simulink model "Simulink_Simulation"  (R2022b)
settings: Solver=FixedStepAuto  StartTime=0.0  StopTime=30  FixedStep=5e-4  RelTol=1e-3
values from neighbouring files (symbols this model uses):
  Kd_PitchRate_val = 2    [Simscape_Simulation_Init.m]
  Kd_RollRate_val = 3    [Simscape_Simulation_Init.m]
  Kd_YawRate_val = 0e6    (= 0)    [Simscape_Simulation_Init.m]
  Ki_PitchRate_val = 7    [Simscape_Simulation_Init.m]
  Ki_RollRate_val = 7    [Simscape_Simulation_Init.m]
  Ki_Thrust_val = 200e6    (= 200000000)    [Simscape_Simulation_Init.m]
  Ki_YawRate_val = 100e6    (= 100000000)    [Simscape_Simulation_Init.m]
  Kp_PitchRate_val = 20    [Simscape_Simulation_Init.m]
  Kp_RollRate_val = 25    [Simscape_Simulation_Init.m]
  Kp_Thrust_val = 2e6    (= 2000000)    [Simscape_Simulation_Init.m]
  Kp_YawRate_val = 110e6    (= 110000000)    [Simscape_Simulation_Init.m]
  Kq_PitchRate_val = 4    [Simscape_Simulation_Init.m]
  Kr_YawRate_val = 7    [Simscape_Simulation_Init.m]
  N_PitchRate_val = 20    [Simscape_Simulation_Init.m]
  N_YawRate_val = 20    [Simscape_Simulation_Init.m]
  Ts_val = 0.01    [Simscape_Simulation_Init.m]
undefined symbols (not defined in the file or in its folder): DiscIntNeverNeededParam, smiData, X, Y, Z
libraries: sm_lib x27, nesl_utility x14, slpidlib x2, simulink x1
(part 1 of 2)
settings Model: Creator=marcv  LastModifiedBy=marcv

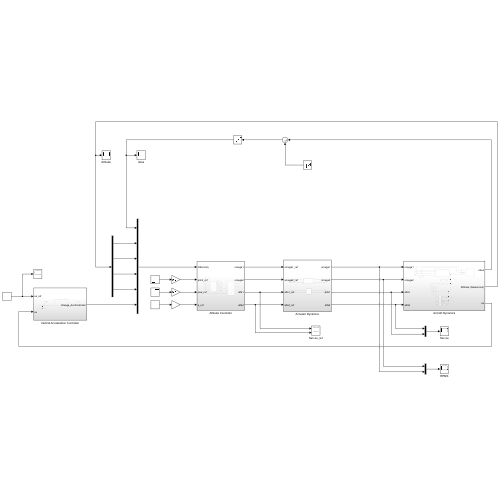
[thumbnail: Simulink's stored preview of the top-level diagram]
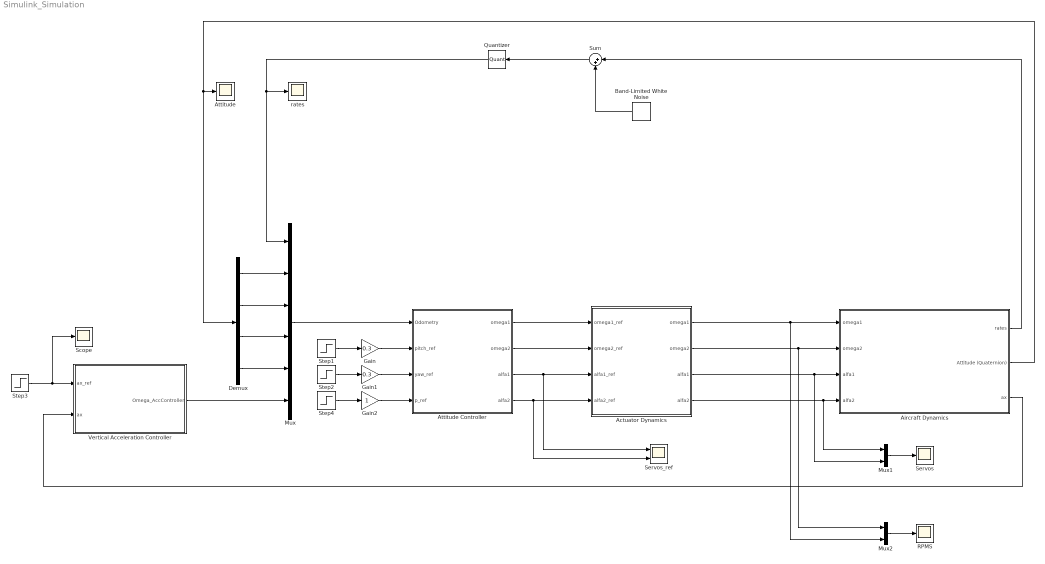
== system Simulink_Simulation ==
  Actuator Dynamics : Subsystem
  Aircraft Dynamics : Subsystem
  Attitude : Scope
  Attitude Controller : Subsystem
  Band-Limited White Noise : simulink/Sources/Band-Limited White Noise  Cov=[1e-6]  Ts=Ts_val  seed=[23341,43241,31231]
  Demux : Demux
  Gain : Gain  Gain=0.3
  Gain1 : Gain  Gain=0.3
  Gain2 : Gain
  Mux : Mux  Inputs=6
  Mux1 : Mux  Inputs=2
  Mux2 : Mux  Inputs=2
  Quantizer : Quantizer  QuantizationInterval=1e-3
  RPMS : Scope
  Scope : Scope
  Servos : Scope
  Servos_ref : Scope  NumInputPorts=2
  Step1 : Step  Time=10  SampleTime=0
  Step2 : Step  Time=10  SampleTime=0
  Step3 : Step  Before=2  After=2  SampleTime=0
  Step4 : Step  Time=10  SampleTime=0
  Sum : Sum  Inputs=|++
  Vertical Acceleration Controller : Subsystem
  rates : Scope
  wires:
  Mux/1 -> Attitude Controller/1(Odometry)
  Aircraft Dynamics/2(Attitude (Quaternion)) -> Demux/1, Attitude/1
  Aircraft Dynamics/3(ax) -> Vertical Acceleration Controller/2(ax)
  Step3/1 -> Scope/1, Vertical Acceleration Controller/1(ax_ref)
  Mux1/1 -> Servos/1
  Mux2/1 -> RPMS/1
  Vertical Acceleration Controller/1(Omega_AccController) -> Mux/6
  Demux/4 -> Mux/5
  Demux/3 -> Mux/4
  Demux/2 -> Mux/3
  Demux/1 -> Mux/2
  Gain/1 -> Attitude Controller/2(pitch_ref)
  Step1/1 -> Gain/1
  Step4/1 -> Gain2/1
  Step2/1 -> Gain1/1
  Gain1/1 -> Attitude Controller/3(yaw_ref)
  Gain2/1 -> Attitude Controller/4(p_ref)
  Actuator Dynamics/2(omega2) -> Aircraft Dynamics/2(omega2), Mux2/1
  Actuator Dynamics/3(alfa1) -> Mux1/2, Aircraft Dynamics/3(alfa1)
  Actuator Dynamics/4(alfa2) -> Mux1/1, Aircraft Dynamics/4(alfa2)
  Actuator Dynamics/1(omega1) -> Mux2/2, Aircraft Dynamics/1(omega1)
  Attitude Controller/1(omega1) -> Actuator Dynamics/1(omega1_ref)
  Attitude Controller/2(omega2) -> Actuator Dynamics/2(omega2_ref)
  Attitude Controller/3(alfa1) -> Actuator Dynamics/3(alfa1_ref), Servos_ref/1
  Attitude Controller/4(alfa2) -> Servos_ref/2, Actuator Dynamics/4(alfa2_ref)
  Quantizer/1 -> rates/1, Mux/1
  Aircraft Dynamics/1(rates) -> Sum/1
  Sum/1 -> Quantizer/1
  Band-Limited White Noise/1 -> Sum/2

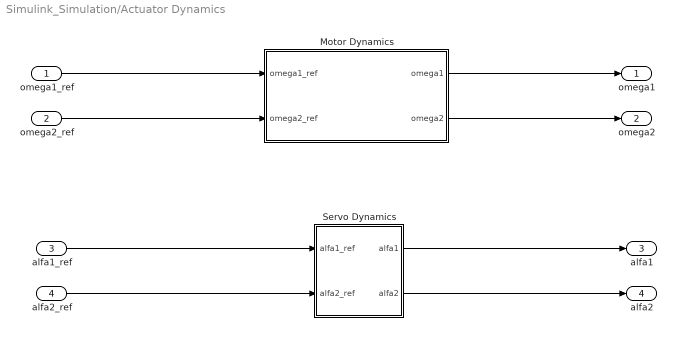
== system Simulink_Simulation/Actuator Dynamics ==
  omega1_ref : Inport
  omega2_ref : Inport  Port=2
  alfa1_ref : Inport  Port=3
  alfa2_ref : Inport  Port=4
  Motor Dynamics : Subsystem
  Servo Dynamics : Subsystem
  omega1 : Outport
  omega2 : Outport  Port=2
  alfa1 : Outport  Port=3
  alfa2 : Outport  Port=4
  wires:
  omega1_ref/1 -> Motor Dynamics/1(omega1_ref)
  alfa2_ref/1 -> Servo Dynamics/2(alfa2_ref)
  alfa1_ref/1 -> Servo Dynamics/1(alfa1_ref)
  omega2_ref/1 -> Motor Dynamics/2(omega2_ref)
  Servo Dynamics/1(alfa1) -> alfa1/1
  Servo Dynamics/2(alfa2) -> alfa2/1
  Motor Dynamics/1(omega1) -> omega1/1
  Motor Dynamics/2(omega2) -> omega2/1

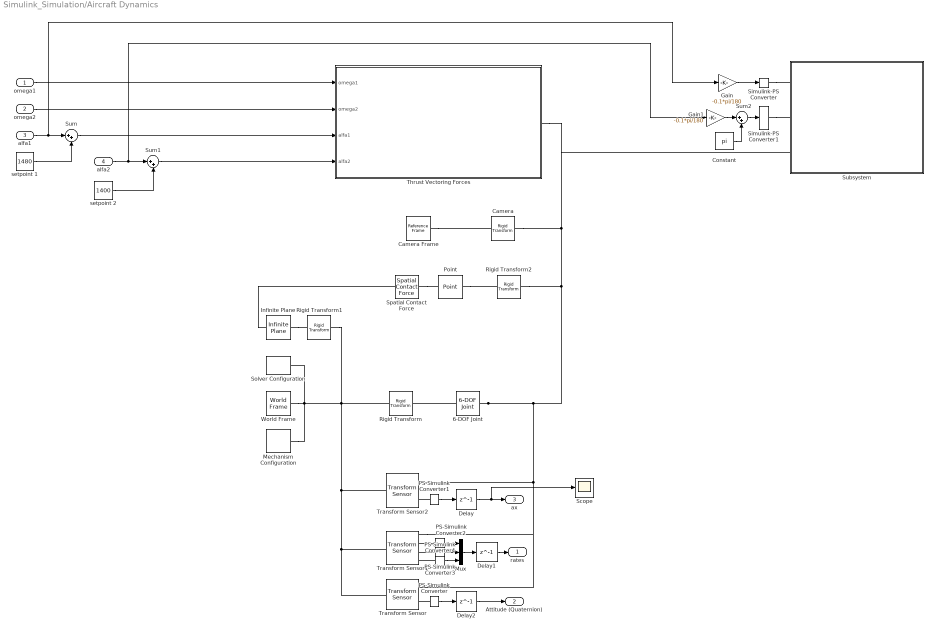
== system Simulink_Simulation/Aircraft Dynamics ==
  omega1 : Inport
  omega2 : Inport  Port=2
  alfa1 : Inport  Port=3
  alfa2 : Inport  Port=4
  6-DOF Joint : sm_lib/Joints/6-DOF Joint  JointMode=Normal  SenseConstraintForce=off  SenseConstraintForceX=off  SenseConstraintForceY=off  SenseConstraintForceZ=off  SenseConstraintTorque=off  SenseConstraintTorqueX=off  SenseConstraintTorqueY=off  SenseConstraintTorqueZ=off  SenseTotalForce=off  SenseTotalForceX=off  SenseTotalForceY=off  SenseTotalForceZ=off  SenseTotalTorque=off  SenseTotalTorqueX=off  SenseTotalTorqueY=off  SenseTotalTorqueZ=off  CompositeWrenchDir=FollowerOnBase  CompositeWrenchFrame=BaseFrame  PxEquilibriumPosition=0  PxEquilibriumPositionUnits=m  PxSpringStiffness=0  PxSpringStiffnessUnits=N/m  PxDampingCoefficient=0  PxDampingCoefficientUnits=N/(m/s)  PxTorqueActuationMode=NoTorque  PxMotionActuationMode=ComputedMotion  PxSensePosition=off  PxSenseVelocity=off  PxSenseAcceleration=off  PxSenseTorqueForce=off  PxSenseLowerLimitTorqueForce=off  PxSenseUpperLimitTorqueForce=off  PxLowerLimitSpecify=off  PxLowerLimitBound=-1  PxLowerLimitBoundUnits=m  PxLowerLimitStiffness=1e6  PxLowerLimitStiffnessUnits=N/m  PxLowerLimitDamping=1e3  PxLowerLimitDampingUnits=N/(m/s)  PxLowerLimitTransitionRegionWidth=1e-4  PxLowerLimitTransitionRegionWidthUnits=m  PxUpperLimitSpecify=off  PxUpperLimitBound=1  PxUpperLimitBoundUnits=m  PxUpperLimitStiffness=1e6  PxUpperLimitStiffnessUnits=N/m  PxUpperLimitDamping=1e3  PxUpperLimitDampingUnits=N/(m/s)  PxUpperLimitTransitionRegionWidth=1e-4  PxUpperLimitTransitionRegionWidthUnits=m  PxPositionTargetSpecify=off  PxPositionTargetPriority=High  PxPositionTargetValue=0  PxPositionTargetValueUnits=m  PxVelocityTargetSpecify=off  PxVelocityTargetPriority=High  PxVelocityTargetValue=0  PxVelocityTargetValueUnits=m/s  PyEquilibriumPosition=0  PyEquilibriumPositionUnits=m  PySpringStiffness=0  PySpringStiffnessUnits=N/m  PyDampingCoefficient=0  PyDampingCoefficientUnits=N/(m/s)  PyTorqueActuationMode=NoTorque  PyMotionActuationMode=ComputedMotion  PySensePosition=off  PySenseVelocity=off  PySenseAcceleration=off  PySenseTorqueForce=off  PySenseLowerLimitTorqueForce=off  PySenseUpperLimitTorqueForce=off  PyLowerLimitSpecify=off  PyLowerLimitBound=-1  PyLowerLimitBoundUnits=m  PyLowerLimitStiffness=1e6  PyLowerLimitStiffnessUnits=N/m  PyLowerLimitDamping=1e3  PyLowerLimitDampingUnits=N/(m/s)  PyLowerLimitTransitionRegionWidth=1e-4  PyLowerLimitTransitionRegionWidthUnits=m  PyUpperLimitSpecify=off  PyUpperLimitBound=1  PyUpperLimitBoundUnits=m  PyUpperLimitStiffness=1e6  PyUpperLimitStiffnessUnits=N/m  PyUpperLimitDamping=1e3  PyUpperLimitDampingUnits=N/(m/s)  PyUpperLimitTransitionRegionWidth=1e-4  PyUpperLimitTransitionRegionWidthUnits=m  PyPositionTargetSpecify=off  PyPositionTargetPriority=High  PyPositionTargetValue=0  PyPositionTargetValueUnits=m  PyVelocityTargetSpecify=off  PyVelocityTargetPriority=High  PyVelocityTargetValue=0  PyVelocityTargetValueUnits=m/s  PzEquilibriumPosition=0  PzEquilibriumPositionUnits=m  PzSpringStiffness=0  PzSpringStiffnessUnits=N/m  PzDampingCoefficient=0  PzDampingCoefficientUnits=N/(m/s)  PzTorqueActuationMode=NoTorque  PzMotionActuationMode=ComputedMotion  PzSensePosition=off  PzSenseVelocity=off  PzSenseAcceleration=off  PzSenseTorqueForce=off  PzSenseLowerLimitTorqueForce=off  PzSenseUpperLimitTorqueForce=off  PzLowerLimitSpecify=off  PzLowerLimitBound=-1  PzLowerLimitBoundUnits=m  PzLowerLimitStiffness=1e6  PzLowerLimitStiffnessUnits=N/m  PzLowerLimitDamping=1e3  PzLowerLimitDampingUnits=N/(m/s)  PzLowerLimitTransitionRegionWidth=1e-4  PzLowerLimitTransitionRegionWidthUnits=m  PzUpperLimitSpecify=off  PzUpperLimitBound=1  PzUpperLimitBoundUnits=m  PzUpperLimitStiffness=1e6  PzUpperLimitStiffnessUnits=N/m  PzUpperLimitDamping=1e3  PzUpperLimitDampingUnits=N/(m/s)  PzUpperLimitTransitionRegionWidth=1e-4  PzUpperLimitTransitionRegionWidthUnits=m  PzPositionTargetSpecify=off  PzPositionTargetPriority=High  PzPositionTargetValue=0  PzPositionTargetValueUnits=m  PzVelocityTargetSpecify=off  PzVelocityTargetPriority=High  PzVelocityTargetValue=0  PzVelocityTargetValueUnits=m/s  SphEqPosRotationMethod=None  SphEqPosRotationAngleUnits=deg  SphEqPosRotationStandardAxis=+Z  SphEqPosRotationAngle=0.0  SphEqPosRotationArbitraryAxis=[0 0 1]  SphEqPosFollAlignAxisA=+X  SphEqPosBaseAlignAxisA=+Y  SphEqPosFollAlignAxisB=+Y  SphEqPosBaseAlignAxisB=+Z  SphEqPosRotationSequenceAxes=FollowerAxes  SphEqPosRotationSequence=XYX  SphEqPosRotationSequenceAngles=[0 0 0]  SphEqPosRotationSequenceAnglesUnits=deg  SphEqPosRotationMatrix=[1 0 0; 0 1 0; 0 0 1]  SphEqPosQuaternion=[1 0 0 0]  SphSpringStiffness=0  SphSpringStiffnessUnits=N*m/deg  SphDampingCoefficient=0  SphDampingCoefficientUnits=N*m/(deg/s)  SphActuateTorqueX=off  SphActuateTorqueY=off  SphActuateTorqueZ=off  SphActuateTorque=off  SphTorqueActuationMode=NoTorque  SphMotionActuationMode=ComputedMotion  SphActuationFrame=BaseFrame  SphSensePosition=off  SphSenseVelocityX=off  SphSenseVelocityY=off  SphSenseVelocityZ=off  SphSenseVelocity=off  SphSenseAccelerationX=off  SphSenseAccelerationY=off  SphSenseAccelerationZ=off  SphSenseAcceleration=off  SphSenseTorqueX=off  SphSenseTorqueY=off  SphSenseTorqueZ=off  SphSenseTorqueForce=off  SphSenseLowerLimitTorqueMag=off  SphSenseUpperLimitTorqueMag=off  SphSensingFrame=BaseFrame  SphLowerLimitSpecify=off  SphLowerLimitBound=15  SphLowerLimitBoundUnits=deg  SphLowerLimitStiffness=1e4  SphLowerLimitStiffnessUnits=N*m/deg  SphLowerLimitDamping=10  SphLowerLimitDampingUnits=N*m/(deg/s)  SphLowerLimitTransitionRegionWidth=0.1  SphLowerLimitTransitionRegionWidthUnits=deg  SphUpperLimitSpecify=off  SphUpperLimitBound=45  SphUpperLimitBoundUnits=deg  SphUpperLimitStiffness=1e4  SphUpperLimitStiffnessUnits=N*m/deg  SphUpperLimitDamping=10  SphUpperLimitDampingUnits=N*m/(deg/s)  SphUpperLimitTransitionRegionWidth=0.1  SphUpperLimitTransitionRegionWidthUnits=deg  SphPositionTargetRotationMethod=None  SphPositionTargetRotationAngleUnits=deg  SphPositionTargetRotationStandardAxis=+Z  SphPositionTargetRotationAngle=0.0  SphPositionTargetRotationArbitraryAxis=[0 0 1]  SphPositionTargetFollAlignAxisA=+X  SphPositionTargetBaseAlignAxisA=+Y  SphPositionTargetFollAlignAxisB=+Y  SphPositionTargetBaseAlignAxisB=+Z  SphPositionTargetRotationSequenceAxes=FollowerAxes  SphPositionTargetRotationSequence=XYX  SphPositionTargetRotationSequenceAngles=[0 0 0]  SphPositionTargetRotationSequenceAnglesUnits=deg  SphPositionTargetRotationMatrix=[1 0 0; 0 1 0; 0 0 1]  SphPositionTargetQuaternion=[1 0 0 0]  SphPositionTargetSpecify=off  SphPositionTargetPriority=High  SphVelocityTargetValue=[0 0 0]  SphVelocityTargetValueUnits=deg/s  SphVelocityTargetSpecify=off  SphVelocityTargetPriority=High  SphVelocityTargetInFollowerFrame=on
  Camera : sm_lib/Frames and Transforms/Rigid Transform  TranslationMethod=Cartesian  TranslationStandardOffset=0  TranslationLengthUnit=m  TranslationStandardAxis=+Z  TranslationCartesianOffset=[1 1 1]  TranslationROffset=0  TranslationROffsetUnits=m  TranslationZOffset=0  TranslationZOffsetUnits=m  TranslationThetaOffset=0  TranslationThetaOffsetUnits=deg  RotationMethod=None  RotationAngleUnits=deg  RotationStandardAxis=+Z  RotationAngle=0.0  RotationArbitraryAxis=[0 0 1]  FollAlignAxisA=+X  BaseAlignAxisA=+Y  FollAlignAxisB=+Y  BaseAlignAxisB=+Z  RotationSequenceAxes=FollowerAxes  RotationSequence=XYX  RotationSequenceAngles=[0 0 0]  RotationSequenceAnglesUnits=deg  RotationMatrix=[1 0 0; 0 1 0; 0 0 1]  Quaternion=[cosd(-45),0,sind(-45),0]
  Camera Frame : sm_lib/Frames and Transforms/Reference Frame
  Constant : Constant  Value=pi
  Delay : Delay  DelayLength=1
  Delay1 : Delay  DelayLength=1
  Delay2 : Delay  DelayLength=1
  Gain : Gain  Gain=-0.1*pi/180
  Gain1 : Gain  Gain=-0.1*pi/180
  Infinite Plane : sm_lib/Curves and Surfaces/Infinite Plane  GraphicType=Rectangle  GraphicPlaneWidth=100  GraphicPlaneWidthUnits=m  GraphicPlaneHeight=100  GraphicPlaneHeightUnits=m  GraphicVisPropType=SimpleVisualProperties  GraphicDiffuseColor=[0.4667 0.6745 0.1882]  GraphicOpacity=0.5  GraphicSpecularColor=[0.5 0.5 0.5 1.0]  GraphicAmbientColor=[0.15 0.15 0.15 1.0]  GraphicEmissiveColor=[0.0 0.0 0.0 1.0]  GraphicShininess=75
  Mechanism Configuration : sm_lib/Utilities/Mechanism Configuration  UniformGravity=Constant  GravityVector=[0 0 -9.81]  GravityUnits=m/s^2  LinearizationDelta=0.001  JointModeTransitionNonlinearIterations=2
  Mux : Mux  Inputs=3
  PS-Simulink Converter{,1..4} (5 alike) : nesl_utility/PS-Simulink Converter  PhysicalDomain=network_engine_domain  SubClassName=ps_output  LeftPortType=input  RightPortType=output  PseudoPeriodic=off  Frequencies=[]  VectorFormat=inherit  Unit=inherit  AffineConversion=off
  Point : sm_lib/Curves and Surfaces/Point  GraphicType=Marker  MarkerShape=Sphere  MarkerSize=5  GraphicVisPropType=SimpleVisualProperties  GraphicDiffuseColor=[0.5 0.5 0.5]  GraphicOpacity=1.0  GraphicSpecularColor=[0.5 0.5 0.5 1.0]  GraphicAmbientColor=[0.15 0.15 0.15 1.0]  GraphicEmissiveColor=[0.0 0.0 0.0 1.0]  GraphicShininess=75
  Rigid Transform : sm_lib/Frames and Transforms/Rigid Transform  TranslationMethod=None  TranslationStandardOffset=0  TranslationLengthUnit=m  TranslationStandardAxis=+Z  TranslationCartesianOffset=[0 0 0]  TranslationROffset=0  TranslationROffsetUnits=m  TranslationZOffset=0  TranslationZOffsetUnits=m  TranslationThetaOffset=0  TranslationThetaOffsetUnits=deg  RotationMethod=Quaternion  RotationAngleUnits=deg  RotationStandardAxis=+Z  RotationAngle=0.0  RotationArbitraryAxis=[0 0 1]  FollAlignAxisA=+X  BaseAlignAxisA=+Y  FollAlignAxisB=+Y  BaseAlignAxisB=+Z  RotationSequenceAxes=FollowerAxes  RotationSequence=XYX  RotationSequenceAngles=[0 0 0]  RotationSequenceAnglesUnits=deg  RotationMatrix=[1 0 0; 0 1 0; 0 0 1]  Quaternion=[cosd(-45),0,sind(-45),0]
  Rigid Transform1 : sm_lib/Frames and Transforms/Rigid Transform  TranslationMethod=Cartesian  TranslationStandardOffset=0  TranslationLengthUnit=m  TranslationStandardAxis=+Z  TranslationCartesianOffset=[0 0 0.035]  TranslationROffset=0  TranslationROffsetUnits=m  TranslationZOffset=0  TranslationZOffsetUnits=m  TranslationThetaOffset=0  TranslationThetaOffsetUnits=deg  RotationMethod=None  RotationAngleUnits=deg  RotationStandardAxis=+Z  RotationAngle=0.0  RotationArbitraryAxis=[0 0 1]  FollAlignAxisA=+X  BaseAlignAxisA=+Y  FollAlignAxisB=+Y  BaseAlignAxisB=+Z  RotationSequenceAxes=FollowerAxes  RotationSequence=XYX  RotationSequenceAngles=[0 0 0]  RotationSequenceAnglesUnits=deg  RotationMatrix=[1 0 0; 0 1 0; 0 0 1]  Quaternion=[cosd(-45),0,sind(-45),0]
  Rigid Transform2 : sm_lib/Frames and Transforms/Rigid Transform  TranslationMethod=Cartesian  TranslationStandardOffset=0  TranslationLengthUnit=m  TranslationStandardAxis=+Z  TranslationCartesianOffset=[0.04 0 0]  TranslationROffset=0  TranslationROffsetUnits=m  TranslationZOffset=0  TranslationZOffsetUnits=m  TranslationThetaOffset=0  TranslationThetaOffsetUnits=deg  RotationMethod=None  RotationAngleUnits=deg  RotationStandardAxis=+Z  RotationAngle=0.0  RotationArbitraryAxis=[0 0 1]  FollAlignAxisA=+X  BaseAlignAxisA=+Y  FollAlignAxisB=+Y  BaseAlignAxisB=+Z  RotationSequenceAxes=FollowerAxes  RotationSequence=XYX  RotationSequenceAngles=[0 0 0]  RotationSequenceAnglesUnits=deg  RotationMatrix=[1 0 0; 0 1 0; 0 0 1]  Quaternion=[cosd(-45),0,sind(-45),0]
  Scope : Scope
  Simulink-PS Converter : nesl_utility/Simulink-PS Converter  PhysicalDomain=network_engine_domain  SubClassName=ps_input  LeftPortType=input  RightPortType=output  PseudoPeriodic=off  Frequencies=[]  NoiseDistribution=none  NoiseParameters=[]  Unit=1  AffineConversion=off  FilteringAndDerivatives=filter  SimscapeFilterOrder=2  InputFilterTimeConstant=0.001  UdotUserProvided=0
  Simulink-PS Converter1 : nesl_utility/Simulink-PS Converter  PhysicalDomain=network_engine_domain  SubClassName=ps_input  LeftPortType=input  RightPortType=output  PseudoPeriodic=off  Frequencies=[]  NoiseDistribution=none  NoiseParameters=[]  Unit=1  AffineConversion=off  FilteringAndDerivatives=filter  SimscapeFilterOrder=2  InputFilterTimeConstant=0.001  UdotUserProvided=0
  Solver Configuration : nesl_utility/Solver Configuration  PhysicalDomain=network_engine_domain  SubClassName=solver  LeftPortType=input  RightPortType=generic  Tones=[]  Harmonics=[]  SimulateNoise=off  Profile=off  UseLocalSampling=off  EnableSwitchedLinearOptims=on  FrequencyDomain=off  UseCCode=off  RelTol=0.001  AbsTol=1e-06  MinStep=1e-09  ToWorkspace=off  RevertToSquareIcSolve=off  NumHomotopyIterations=100  PhasorMode=off  PhasorModeNumHarmonics=1  ConsistencySolver=NEWTON_XTOL_AFTER_FTOL  IndexReductionMethod=DerivativeReplacement  DoDC=off  ResidualTolerance=1e-09  ConsistencyTolSource=GLOBAL  ConsistencyAbsTol=0.001  ConsistencyRelTol=0.001  ConsistencyTolFactor=0.001  UseLocalSolver=off  LocalSolverChoice=NE_BACKWARD_EULER_ADVANCER  ResolveIndetEquations=on  FunctionEvalNumThread=1  LocalSolverSampleTime=0.001  DoFixedCost=off  MaxNonlinIter=3  MaxModeIter=2  ComputeImpulses=off  ImpulseIterations=2  LinearAlgebra=Sparse  LinearAlgebraNumThread=0  EquationFormulation=NE_TIME_EF  DelaysMemoryBudget=1024  AutomaticFiltering=on  FilteringTimeConstant=0.001  PartitionStorageMethod=AS_NEEDED  PartitionMemoryBudget=1024  PartitionMethod=FAST
  Spatial Contact Force : sm_lib/Forces and Torques/Spatial Contact Force  SenseContactBaseRotation=off  SenseContactBaseTranslation=off  CoefficientOfDynamicFriction=0.3  CoefficientOfStaticFriction=4  NormalDamping=20  NormalDampingUnits=N/(m/s)  SenseContactSignal=off  NormalStiffness=1e3  NormalStiffnessUnits=N/m  FrictionalCriticalVelocity=1e-3  FrictionalCriticalVelocityUnits=m/s  ZeroCrossDetectContactStartAndEnd=off  SenseContactFollowerRotation=off  SenseContactFollowerTranslation=off  FrictionType=SmoothStickSlip  SenseFrictionalForceMagnitude=off  SenseNormalForceMagnitude=off  NormalForceType=SmoothSpringDamper  SenseNormalVelocity=off  SenseSeparationDistance=off  SenseTangentialVelocity=off  NormalTransitionRegionWidth=1e-4  NormalTransitionRegionWidthUnits=m
  Subsystem : Subsystem
  Sum : Sum  Inputs=|++
  Sum1 : Sum  Inputs=|++
  Sum2 : Sum  Inputs=|++
  Thrust Vectoring Forces : Subsystem
  Transform Sensor : sm_lib/Frames and Transforms/Transform Sensor  MeasurementFrame=World  SenseAngle=off  SenseAxis=off  SenseQ=on  SenseR=off  SenseRotationSequence=off  RotationSequence=XYX  SenseOmegaX=off  SenseOmegaY=off  SenseOmegaZ=off  SenseQDot=off  SenseRDot=off  SenseAlphaX=off  SenseAlphaY=off  SenseAlphaZ=off  SenseQDDot=off  SenseRDDot=off  SenseX=off  SenseY=off  SenseZ=off  SenseRad=off  SenseAzim=off  SenseDist=off  SenseInc=off  SenseXDot=off  SenseYDot=off  SenseZDot=off  SenseRadDot=off  SenseAzimDot=off  SenseDistDot=off  SenseIncDot=off  SenseXDDot=off  SenseYDDot=off  SenseZDDot=off  SenseRadDDot=off  SenseAzimDDot=off  SenseDistDDot=off  SenseIncDDot=off
  Transform Sensor1 : sm_lib/Frames and Transforms/Transform Sensor  MeasurementFrame=NonRotatingFollower  SenseAngle=off  SenseAxis=off  SenseQ=off  SenseR=off  SenseRotationSequence=off  RotationSequence=XYX  SenseOmegaX=on  SenseOmegaY=on  SenseOmegaZ=on  SenseQDot=off  SenseRDot=off  SenseAlphaX=off  SenseAlphaY=off  SenseAlphaZ=off  SenseQDDot=off  SenseRDDot=off  SenseX=off  SenseY=off  SenseZ=off  SenseRad=off  SenseAzim=off  SenseDist=off  SenseInc=off  SenseXDot=off  SenseYDot=off  SenseZDot=off  SenseRadDot=off  SenseAzimDot=off  SenseDistDot=off  SenseIncDot=off  SenseXDDot=off  SenseYDDot=off  SenseZDDot=off  SenseRadDDot=off  SenseAzimDDot=off  SenseDistDDot=off  SenseIncDDot=off
  Transform Sensor2 : sm_lib/Frames and Transforms/Transform Sensor  MeasurementFrame=NonRotatingFollower  SenseAngle=off  SenseAxis=off  SenseQ=off  SenseR=off  SenseRotationSequence=off  RotationSequence=XYX  SenseOmegaX=off  SenseOmegaY=off  SenseOmegaZ=off  SenseQDot=off  SenseRDot=off  SenseAlphaX=off  SenseAlphaY=off  SenseAlphaZ=off  SenseQDDot=off  SenseRDDot=off  SenseX=off  SenseY=off  SenseZ=off  SenseRad=off  SenseAzim=off  SenseDist=off  SenseInc=off  SenseXDot=off  SenseYDot=off  SenseZDot=off  SenseRadDot=off  SenseAzimDot=off  SenseDistDot=off  SenseIncDot=off  SenseXDDot=on  SenseYDDot=off  SenseZDDot=off  SenseRadDDot=off  SenseAzimDDot=off  SenseDistDDot=off  SenseIncDDot=off
  World Frame : sm_lib/Frames and Transforms/World Frame
  setpoint 1 : Constant  Value=1480
  setpoint 2 : Constant  Value=1400
  rates : Outport
  Attitude (Quaternion) : Outport  Port=2
  ax : Outport  Port=3
  wires:
  PS-Simulink Converter/1 -> Delay2/1
  PS-Simulink Converter1/1 -> Delay/1
  PS-Simulink Converter2/1 -> Mux/1
  Delay/1 -> Scope/1, ax/1
  Delay2/1 -> Attitude (Quaternion)/1
  omega1/1 -> Thrust Vectoring Forces/1(omega1)
  omega2/1 -> Thrust Vectoring Forces/2(omega2)
  setpoint 1/1 -> Sum/2
  Sum/1 -> Thrust Vectoring Forces/3(alfa1)
  alfa1/1 -> Gain/1, Sum/1
  alfa2/1 -> Sum1/1, Gain1/1
  setpoint 2/1 -> Sum1/2
  Sum1/1 -> Thrust Vectoring Forces/4(alfa2)
  Gain/1 -> Simulink-PS Converter/1
  Gain1/1 -> Sum2/1
  Sum2/1 -> Simulink-PS Converter1/1
  Constant/1 -> Sum2/2
  Delay1/1 -> rates/1
  PS-Simulink Converter4/1 -> Mux/3
  PS-Simulink Converter3/1 -> Mux/2
  Mux/1 -> Delay1/1
  connections:
  6-DOF Joint/RConn1 -- Camera/LConn1 -- Thrust Vectoring Forces/RConn1 -- Subsystem/LConn3 -- Rigid Transform2/LConn1 -- Transform Sensor2/RConn1 -- Transform Sensor/RConn1 -- Transform Sensor1/RConn1
  Transform Sensor/LConn1 -- Transform Sensor2/LConn1 -- Rigid Transform1/LConn1 -- Rigid Transform/LConn1 -- World Frame/RConn1 -- Solver Configuration/RConn1 -- Mechanism Configuration/RConn1 -- Transform Sensor1/LConn1
  PS-Simulink Converter/LConn1 -- Transform Sensor/RConn2
  6-DOF Joint/LConn1 -- Rigid Transform/RConn1
  PS-Simulink Converter1/LConn1 -- Transform Sensor2/RConn2
  Simulink-PS Converter/RConn1 -- Subsystem/LConn1
  Simulink-PS Converter1/RConn1 -- Subsystem/LConn2
  Spatial Contact Force/LConn1 -- Infinite Plane/RConn1
  Spatial Contact Force/RConn1 -- Point/RConn1
  Point/LConn1 -- Rigid Transform2/RConn1
  PS-Simulink Converter2/LConn1 -- Transform Sensor1/RConn2
  Infinite Plane/LConn1 -- Rigid Transform1/RConn1
  PS-Simulink Converter4/LConn1 -- Transform Sensor1/RConn4
  Transform Sensor1/RConn3 -- PS-Simulink Converter3/LConn1
  Camera Frame/RConn1 -- Camera/RConn1

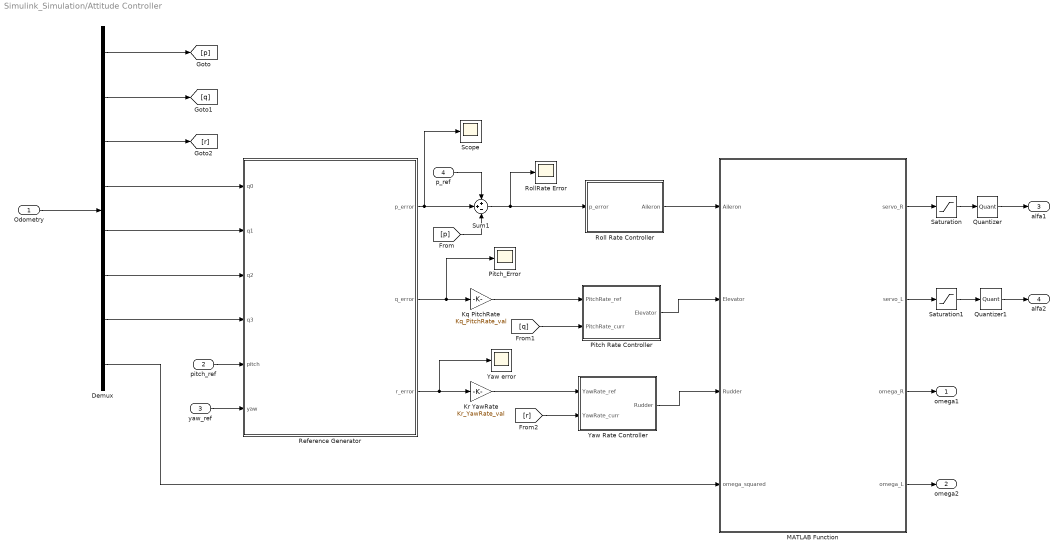
== system Simulink_Simulation/Attitude Controller ==
  Odometry : Inport
  pitch_ref : Inport  Port=2
  yaw_ref : Inport  Port=3
  p_ref : Inport  Port=4
  Demux : Demux  Outputs=8
  Kq PitchRate : Gain  Gain=Kq_PitchRate_val
  Kr YawRate : Gain  Gain=Kr_YawRate_val
  MATLAB Function : MATLAB Function  TreatAsAtomicUnit=on
  Pitch Rate Controller : Subsystem
  Pitch_Error : Scope
  Quantizer : Quantizer  QuantizationInterval=1
  Quantizer1 : Quantizer  QuantizationInterval=1
  Reference Generator : MATLAB Function  TreatAsAtomicUnit=on
  Roll Rate Controller : Subsystem
  RollRate Error : Scope
  Saturation : Saturate  UpperLimit=200  LowerLimit=-200
  Saturation1 : Saturate  UpperLimit=200  LowerLimit=-200
  Scope : Scope
  Sum1 : Sum  Inputs=++-
  Yaw Rate Controller : Subsystem
  Yaw error : Scope
  omega1 : Outport
  omega2 : Outport  Port=2
  alfa1 : Outport  Port=3
  alfa2 : Outport  Port=4
  wires:
  pitch_ref/1 -> Reference Generator/5(pitch)
  yaw_ref/1 -> Reference Generator/6(yaw)
  Odometry/1 -> Demux/1
  Pitch Rate Controller/1(Elevator) -> MATLAB Function/2(Elevator)
  MATLAB Function/1(servo_R) -> Saturation/1
  MATLAB Function/2(servo_L) -> Saturation1/1
  MATLAB Function/4(omega_L) -> omega2/1
  MATLAB Function/3(omega_R) -> omega1/1
  Reference Generator/1(p_error) -> Sum1/2, Scope/1
  Roll Rate Controller/1(Aileron) -> MATLAB Function/1(Aileron)
  Sum1/1 -> RollRate Error/1, Roll Rate Controller/1(p_error)
  Yaw Rate Controller/1(Rudder) -> MATLAB Function/3(Rudder)
  Demux/1 -> [p]
  p_ref/1 -> Sum1/1
  [p] -> Sum1/3
  Reference Generator/2(q_error) -> Pitch_Error/1, Kq PitchRate/1
  Kq PitchRate/1 -> Pitch Rate Controller/1(PitchRate_ref)
  Demux/2 -> [q]
  Demux/3 -> [r]
  Demux/8 -> MATLAB Function/4(omega_squared)
  Demux/7 -> Reference Generator/4(q3)
  Demux/6 -> Reference Generator/3(q2)
  Demux/5 -> Reference Generator/2(q1)
  Demux/4 -> Reference Generator/1(q0)
  Kr YawRate/1 -> Yaw Rate Controller/1(YawRate_ref)
  Reference Generator/3(r_error) -> Yaw error/1, Kr YawRate/1
  Saturation/1 -> Quantizer/1
  Saturation1/1 -> Quantizer1/1
  Quantizer/1 -> alfa1/1
  Quantizer1/1 -> alfa2/1
  [q] -> Pitch Rate Controller/2(PitchRate_curr)
  [r] -> Yaw Rate Controller/2(YawRate_curr)

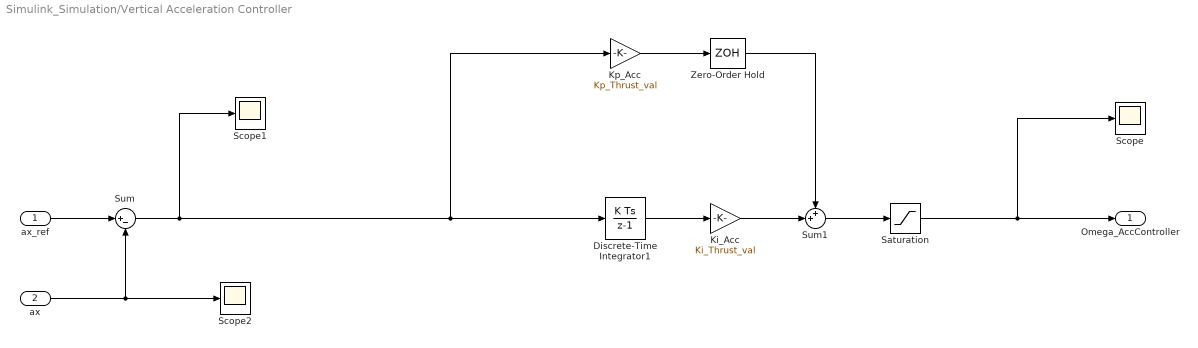
== system Simulink_Simulation/Vertical Acceleration Controller ==
  ax_ref : Inport
  ax : Inport  Port=2
  Discrete-Time Integrator1 : DiscreteIntegrator  SampleTime=Ts_val  ICPrevOutput=DiscIntNeverNeededParam  ICPrevScaledInput=DiscIntNeverNeededParam
  Ki_Acc : Gain  Gain=Ki_Thrust_val
  Kp_Acc : Gain  Gain=Kp_Thrust_val
  Saturation : Saturate  UpperLimit=Inf  LowerLimit=0
  Scope : Scope
  Scope1 : Scope
  Scope2 : Scope
  Sum : Sum  Inputs=|+-
  Sum1 : Sum  Inputs=++|
  Zero-Order Hold : ZeroOrderHold  SampleTime=Ts_val
  Omega_AccController : Outport
  wires:
  ax_ref/1 -> Sum/1
  ax/1 -> Scope2/1, Sum/2
  Discrete-Time Integrator1/1 -> Ki_Acc/1
  Sum/1 -> Kp_Acc/1, Discrete-Time Integrator1/1, Scope1/1
  Ki_Acc/1 -> Sum1/2
  Kp_Acc/1 -> Zero-Order Hold/1
  Zero-Order Hold/1 -> Sum1/1
  Sum1/1 -> Saturation/1
  Saturation/1 -> Scope/1, Omega_AccController/1

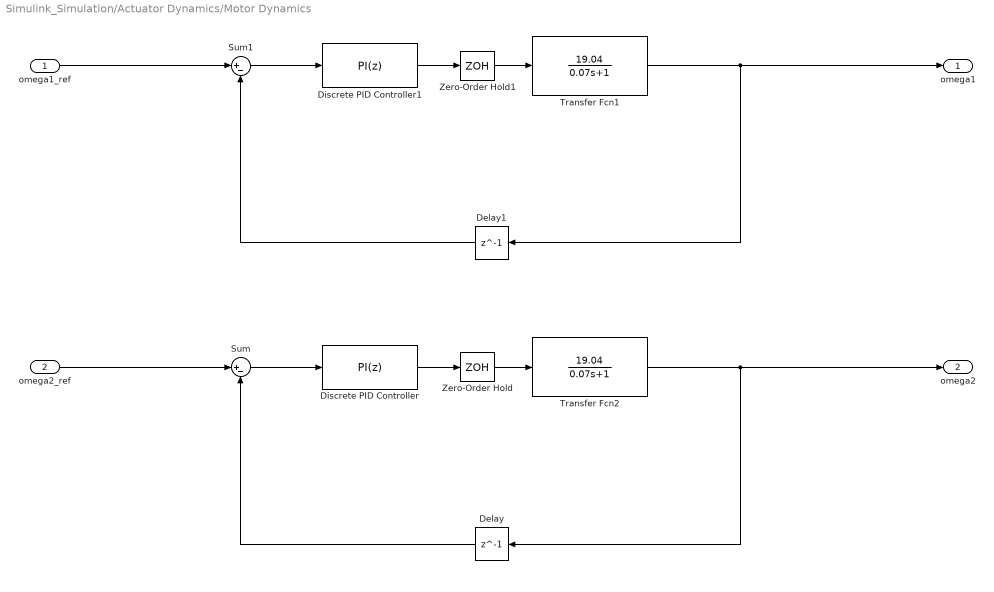
== system Simulink_Simulation/Actuator Dynamics/Motor Dynamics ==
  omega1_ref : Inport
  omega2_ref : Inport  Port=2
  Delay : Delay  DelayLength=1  SampleTime=0.0005
  Delay1 : Delay  DelayLength=1  SampleTime=0.0005
  Discrete PID Controller : slpidlib/PID Controller  Controller=PI  Form=Parallel  TimeDomain=Discrete-time  UseExternalTs=off  SampleTime=0.0005  IntegratorMethod=Forward Euler  FilterMethod=Forward Euler  ControllerParametersSource=internal  P=0.25  I=3  UseKiTs=off  D=0  N=100  UseFilter=on  TunerSelectOption=Transfer Function Based (PID Tuner App)  InitialConditionSource=internal  InitialConditionForIntegrator=0  InitialConditionForFilter=0  DifferentiatorICPrevScaledInput=0  ExternalReset=none  TrackingMode=off  Kt=1  LimitOutput=off  SatLimitsSource=internal  UpperSaturationLimit=inf  LowerSaturationLimit=-inf  LinearizeAsGain=off  AntiWindupMode=none  Kb=1  LimitIntegrator=off  UpperIntegratorSaturationLimit=inf  LowerIntegratorSaturationLimit=-inf  POutMin=[]  POutMax=[]  IOutMin=[]  IOutMax=[]  DOutMin=[]  DOutMax=[]  NOutMin=[]  NOutMax=[]  SumOutMin=[]  SumOutMax=[]  SaturationOutMin=[]  SaturationOutMax=[]  PParamMin=[]  PParamMax=[]  IParamMin=[]  IParamMax=[]  DParamMin=[]  DParamMax=[]  NParamMin=[]  NParamMax=[]  KbParamMin=[]  KbParamMax=[]  KtParamMin=[]  KtParamMax=[]  KbOutMin=[]  KbOutMax=[]  KtOutMin=[]  KtOutMax=[]  IntegratorOutMin=[]  IntegratorOutMax=[]  FilterOutMin=[]  FilterOutMax=[]  SumI1OutMin=[]  SumI1OutMax=[]  SumI2OutMin=[]  SumI2OutMax=[]  SumI3OutMin=[]  SumI3OutMax=[]  SumI4OutMin=[]  SumI4OutMax=[]  SumDOutMin=[]  SumDOutMax=[]  DifferentiatorOutMin=[]  DifferentiatorOutMax=[]  FilterDiffOutCoefMin=[]  FilterDiffOutCoefMax=[]  ReciprocalOutMin=[]  ReciprocalOutMax=[]  SumDenOutMin=[]  SumDenOutMax=[]  SumNumOutMin=[]  SumNumOutMax=[]  DivideOutMin=[]  DivideOutMax=[]  UdiffTsProdOutMin=[]  UdiffTsProdOutMax=[]  NTsProdOutMin=[]  NTsProdOutMax=[]  UintegralTsProdOutMin=[]  UintegralTsProdOutMax=[]  UngainTsProdOutMin=[]  UngainTsProdOutMax=[]  ClampingZeroOutDataTypeStr=Inherit: Inherit via back propagation  ClampingZeroOutMin=[]  ClampingZeroOutMax=[]  FilterDenConstantOutDataTypeStr=Inherit: Inherit via back propagation  FilterDenConstantOutMin=[]  FilterDenConstantOutMax=[]  PCopyOutDataTypeStr=Inherit: Inherit via back propagation  PCopyOutMin=[]  PCopyOutMax=[]  NCopyOutDataTypeStr=Inherit: Inherit via back propagation  NCopyOutMin=[]  NCopyOutMax=[]  IntegratorContinuousStateAttributes=''  IntegratorStateMustResolveToSignalObject=off  IntegratorRTWStateStorageClass=Auto  FilterContinuousStateAttributes=''  FilterStateMustResolveToSignalObject=off  FilterRTWStateStorageClass=Auto  ParallelPVariant=InternalParameters  IdealPVariant=Disabled  IVariant=InternalParameters  DVariant=Disabled  IntegratorVariant=Discrete  SatVariant=Disabled  AWVariant=Passthrough  PCopyVariant=Disabled  TRVariant=Disabled  FdbkBlocksVariant=Forward  IdealPFdbkVariant=Disabled  SatFdbkVariant=Disabled  DerivativeFilterVariant=Disabled  NVariant=Disabled  NCopyVariant=Disabled_SignalSpec  FilterICVariant=Disabled  IntegratorICVariant=InternalICs  ExternalResetVariant=Disabled  TRSumVariant=Passthrough  SumFdbkVariant=Disabled  SumVariant=Sum_PI  TsampFilterVariant=InternalTs  TsampNgainVariant=Passthrough  TsampIntegralVariant=Passthrough  ExternalSaturationOutDataTypeStr=Inherit: Same as second input
      settings: LibrarySourceBlock=simulink/Discrete/Discrete PID Controller
  Discrete PID Controller1 : slpidlib/PID Controller  Controller=PI  Form=Parallel  TimeDomain=Discrete-time  UseExternalTs=off  SampleTime=0.0005  IntegratorMethod=Forward Euler  FilterMethod=Forward Euler  ControllerParametersSource=internal  P=0.25  I=3  UseKiTs=off  D=0  N=100  UseFilter=on  TunerSelectOption=Transfer Function Based (PID Tuner App)  InitialConditionSource=internal  InitialConditionForIntegrator=0  InitialConditionForFilter=0  DifferentiatorICPrevScaledInput=0  ExternalReset=none  TrackingMode=off  Kt=1  LimitOutput=off  SatLimitsSource=internal  UpperSaturationLimit=inf  LowerSaturationLimit=-inf  LinearizeAsGain=off  AntiWindupMode=none  Kb=1  LimitIntegrator=off  UpperIntegratorSaturationLimit=inf  LowerIntegratorSaturationLimit=-inf  POutMin=[]  POutMax=[]  IOutMin=[]  IOutMax=[]  DOutMin=[]  DOutMax=[]  NOutMin=[]  NOutMax=[]  SumOutMin=[]  SumOutMax=[]  SaturationOutMin=[]  SaturationOutMax=[]  PParamMin=[]  PParamMax=[]  IParamMin=[]  IParamMax=[]  DParamMin=[]  DParamMax=[]  NParamMin=[]  NParamMax=[]  KbParamMin=[]  KbParamMax=[]  KtParamMin=[]  KtParamMax=[]  KbOutMin=[]  KbOutMax=[]  KtOutMin=[]  KtOutMax=[]  IntegratorOutMin=[]  IntegratorOutMax=[]  FilterOutMin=[]  FilterOutMax=[]  SumI1OutMin=[]  SumI1OutMax=[]  SumI2OutMin=[]  SumI2OutMax=[]  SumI3OutMin=[]  SumI3OutMax=[]  SumI4OutMin=[]  SumI4OutMax=[]  SumDOutMin=[]  SumDOutMax=[]  DifferentiatorOutMin=[]  DifferentiatorOutMax=[]  FilterDiffOutCoefMin=[]  FilterDiffOutCoefMax=[]  ReciprocalOutMin=[]  ReciprocalOutMax=[]  SumDenOutMin=[]  SumDenOutMax=[]  SumNumOutMin=[]  SumNumOutMax=[]  DivideOutMin=[]  DivideOutMax=[]  UdiffTsProdOutMin=[]  UdiffTsProdOutMax=[]  NTsProdOutMin=[]  NTsProdOutMax=[]  UintegralTsProdOutMin=[]  UintegralTsProdOutMax=[]  UngainTsProdOutMin=[]  UngainTsProdOutMax=[]  ClampingZeroOutDataTypeStr=Inherit: Inherit via back propagation  ClampingZeroOutMin=[]  ClampingZeroOutMax=[]  FilterDenConstantOutDataTypeStr=Inherit: Inherit via back propagation  FilterDenConstantOutMin=[]  FilterDenConstantOutMax=[]  PCopyOutDataTypeStr=Inherit: Inherit via back propagation  PCopyOutMin=[]  PCopyOutMax=[]  NCopyOutDataTypeStr=Inherit: Inherit via back propagation  NCopyOutMin=[]  NCopyOutMax=[]  IntegratorContinuousStateAttributes=''  IntegratorStateMustResolveToSignalObject=off  IntegratorRTWStateStorageClass=Auto  FilterContinuousStateAttributes=''  FilterStateMustResolveToSignalObject=off  FilterRTWStateStorageClass=Auto  ParallelPVariant=InternalParameters  IdealPVariant=Disabled  IVariant=InternalParameters  DVariant=Disabled  IntegratorVariant=Discrete  SatVariant=Disabled  AWVariant=Passthrough  PCopyVariant=Disabled  TRVariant=Disabled  FdbkBlocksVariant=Forward  IdealPFdbkVariant=Disabled  SatFdbkVariant=Disabled  DerivativeFilterVariant=Disabled  NVariant=Disabled  NCopyVariant=Disabled_SignalSpec  FilterICVariant=Disabled  IntegratorICVariant=InternalICs  ExternalResetVariant=Disabled  TRSumVariant=Passthrough  SumFdbkVariant=Disabled  SumVariant=Sum_PI  TsampFilterVariant=InternalTs  TsampNgainVariant=Passthrough  TsampIntegralVariant=Passthrough  ExternalSaturationOutDataTypeStr=Inherit: Same as second input
      settings: LibrarySourceBlock=simulink/Discrete/Discrete PID Controller
  Sum : Sum  Inputs=|+-
  Sum1 : Sum  Inputs=|+-
  Transfer Fcn1 : TransferFcn  Numerator=[19.04]  Denominator=[0.07 1]
  Transfer Fcn2 : TransferFcn  Numerator=[19.04]  Denominator=[0.07 1]
  Zero-Order Hold : ZeroOrderHold  SampleTime=0.0005
  Zero-Order Hold1 : ZeroOrderHold  SampleTime=0.0005
  omega1 : Outport
  omega2 : Outport  Port=2
  wires:
  omega2_ref/1 -> Sum/1
  Delay/1 -> Sum/2
  Zero-Order Hold/1 -> Transfer Fcn2/1
  Transfer Fcn2/1 -> Delay/1, omega2/1
  Discrete PID Controller/1 -> Zero-Order Hold/1
  Sum/1 -> Discrete PID Controller/1
  omega1_ref/1 -> Sum1/1
  Delay1/1 -> Sum1/2
  Discrete PID Controller1/1 -> Zero-Order Hold1/1
  Zero-Order Hold1/1 -> Transfer Fcn1/1
  Sum1/1 -> Discrete PID Controller1/1
  Transfer Fcn1/1 -> omega1/1, Delay1/1

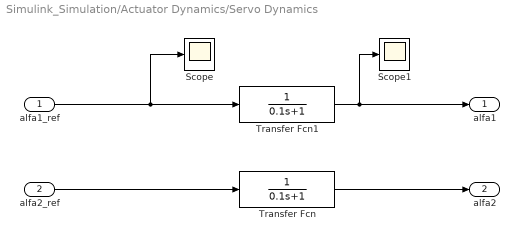
== system Simulink_Simulation/Actuator Dynamics/Servo Dynamics ==
  alfa1_ref : Inport
  alfa2_ref : Inport  Port=2
  Scope : Scope
  Scope1 : Scope
  Transfer Fcn : TransferFcn  Denominator=[0.1 1]
  Transfer Fcn1 : TransferFcn  Denominator=[0.1 1]
  alfa1 : Outport
  alfa2 : Outport  Port=2
  wires:
  Transfer Fcn/1 -> alfa2/1
  Transfer Fcn1/1 -> Scope1/1, alfa1/1
  alfa1_ref/1 -> Transfer Fcn1/1, Scope/1
  alfa2_ref/1 -> Transfer Fcn/1

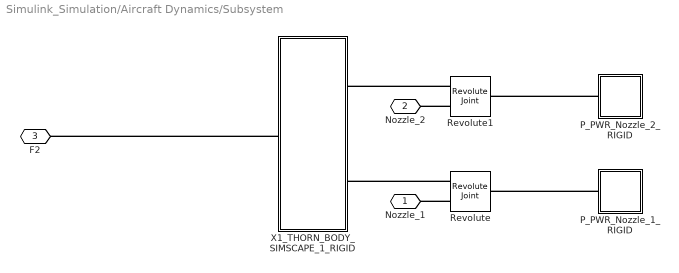
== system Simulink_Simulation/Aircraft Dynamics/Subsystem ==
  P_PWR_Nozzle_1_RIGID : Subsystem
  P_PWR_Nozzle_2_RIGID : Subsystem
  Revolute : sm_lib/Joints/Revolute Joint  JointMode=Normal  SenseConstraintForce=off  SenseConstraintForceX=off  SenseConstraintForceY=off  SenseConstraintForceZ=off  SenseConstraintTorque=off  SenseConstraintTorqueX=off  SenseConstraintTorqueY=off  SenseConstraintTorqueZ=off  SenseTotalForce=off  SenseTotalForceX=off  SenseTotalForceY=off  SenseTotalForceZ=off  SenseTotalTorque=off  SenseTotalTorqueX=off  SenseTotalTorqueY=off  SenseTotalTorqueZ=off  CompositeWrenchDir=FollowerOnBase  CompositeWrenchFrame=BaseFrame  EquilibriumPosition=0  EquilibriumPositionUnits=deg  SpringStiffness=0  SpringStiffnessUnits=N*m/deg  DampingCoefficient=0  DampingCoefficientUnits=N*m/(deg/s)  TorqueActuationMode=ComputedTorque  MotionActuationMode=InputMotion  SensePosition=off  SenseVelocity=off  SenseAcceleration=off  SenseTorqueForce=off  SenseLowerLimitTorqueForce=off  SenseUpperLimitTorqueForce=off  LowerLimitSpecify=off  LowerLimitBound=-90  LowerLimitBoundUnits=deg  LowerLimitStiffness=1e4  LowerLimitStiffnessUnits=N*m/deg  LowerLimitDamping=10  LowerLimitDampingUnits=N*m/(deg/s)  LowerLimitTransitionRegionWidth=0.1  LowerLimitTransitionRegionWidthUnits=deg  UpperLimitSpecify=off  UpperLimitBound=90  UpperLimitBoundUnits=deg  UpperLimitStiffness=1e4  UpperLimitStiffnessUnits=N*m/deg  UpperLimitDamping=10  UpperLimitDampingUnits=N*m/(deg/s)  UpperLimitTransitionRegionWidth=0.1  UpperLimitTransitionRegionWidthUnits=deg  PositionTargetSpecify=on  PositionTargetPriority=Low  PositionTargetValue=smiData.RevoluteJoint(1).Rz.Pos  PositionTargetValueUnits=deg  VelocityTargetSpecify=off  VelocityTargetPriority=High  VelocityTargetValue=0  VelocityTargetValueUnits=deg/s
  Revolute1 : sm_lib/Joints/Revolute Joint  JointMode=Normal  SenseConstraintForce=off  SenseConstraintForceX=off  SenseConstraintForceY=off  SenseConstraintForceZ=off  SenseConstraintTorque=off  SenseConstraintTorqueX=off  SenseConstraintTorqueY=off  SenseConstraintTorqueZ=off  SenseTotalForce=off  SenseTotalForceX=off  SenseTotalForceY=off  SenseTotalForceZ=off  SenseTotalTorque=off  SenseTotalTorqueX=off  SenseTotalTorqueY=off  SenseTotalTorqueZ=off  CompositeWrenchDir=FollowerOnBase  CompositeWrenchFrame=BaseFrame  EquilibriumPosition=0  EquilibriumPositionUnits=deg  SpringStiffness=0  SpringStiffnessUnits=N*m/deg  DampingCoefficient=0  DampingCoefficientUnits=N*m/(deg/s)  TorqueActuationMode=ComputedTorque  MotionActuationMode=InputMotion  SensePosition=off  SenseVelocity=off  SenseAcceleration=off  SenseTorqueForce=off  SenseLowerLimitTorqueForce=off  SenseUpperLimitTorqueForce=off  LowerLimitSpecify=off  LowerLimitBound=-90  LowerLimitBoundUnits=deg  LowerLimitStiffness=1e4  LowerLimitStiffnessUnits=N*m/deg  LowerLimitDamping=10  LowerLimitDampingUnits=N*m/(deg/s)  LowerLimitTransitionRegionWidth=0.1  LowerLimitTransitionRegionWidthUnits=deg  UpperLimitSpecify=off  UpperLimitBound=90  UpperLimitBoundUnits=deg  UpperLimitStiffness=1e4  UpperLimitStiffnessUnits=N*m/deg  UpperLimitDamping=10  UpperLimitDampingUnits=N*m/(deg/s)  UpperLimitTransitionRegionWidth=0.1  UpperLimitTransitionRegionWidthUnits=deg  PositionTargetSpecify=on  PositionTargetPriority=Low  PositionTargetValue=smiData.RevoluteJoint(2).Rz.Pos  PositionTargetValueUnits=deg  VelocityTargetSpecify=off  VelocityTargetPriority=High  VelocityTargetValue=0  VelocityTargetValueUnits=deg/s
  X1_THORN_BODY_SIMSCAPE_1_RIGID : Subsystem
  Nozzle_1 : PMIOPort  Side=Left
  Nozzle_2 : PMIOPort  Port=2  Side=Left
  F2 : PMIOPort  Port=3  Side=Left
  connections:
  Revolute1/LConn1 -- X1_THORN_BODY_SIMSCAPE_1_RIGID/RConn1
  P_PWR_Nozzle_1_RIGID/LConn1 -- Revolute/RConn1
  P_PWR_Nozzle_2_RIGID/LConn1 -- Revolute1/RConn1
  X1_THORN_BODY_SIMSCAPE_1_RIGID/LConn1 -- F2/RConn1
  Revolute/LConn1 -- X1_THORN_BODY_SIMSCAPE_1_RIGID/RConn2
  Revolute1/LConn2 -- Nozzle_2/RConn1
  Revolute/LConn2 -- Nozzle_1/RConn1

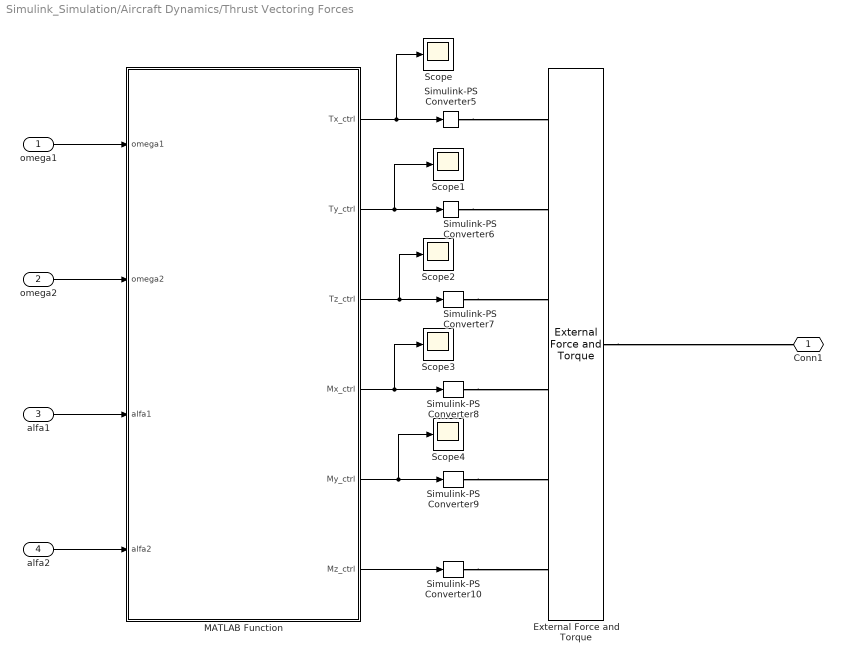
== system Simulink_Simulation/Aircraft Dynamics/Thrust Vectoring Forces ==
  omega1 : Inport
  omega2 : Inport  Port=2
  alfa1 : Inport  Port=3
  alfa2 : Inport  Port=4
  External Force and Torque : sm_lib/Forces and Torques/External Force and Torque  ForceResolutionFrame=AttachedFrame  EnableForceX=on  EnableForceY=on  EnableForceZ=on  EnableForce=off  TorqueResolutionFrame=AttachedFrame  EnableTorqueX=on  EnableTorqueY=on  EnableTorqueZ=on  EnableTorque=off
  MATLAB Function : MATLAB Function  TreatAsAtomicUnit=on
  Scope{,1..4} (5 alike) : Scope
  Simulink-PS Converter{5..10} (6 alike) : nesl_utility/Simulink-PS Converter  PhysicalDomain=network_engine_domain  SubClassName=ps_input  LeftPortType=input  RightPortType=output  PseudoPeriodic=off  Frequencies=[]  NoiseDistribution=none  NoiseParameters=[]  Unit=1  AffineConversion=off  FilteringAndDerivatives=provide  SimscapeFilterOrder=1  InputFilterTimeConstant=0.001  UdotUserProvided=0
  Conn1 : PMIOPort  Side=Right
  wires:
  MATLAB Function/1(Tx_ctrl) -> Scope/1, Simulink-PS Converter5/1
  MATLAB Function/2(Ty_ctrl) -> Scope1/1, Simulink-PS Converter6/1
  MATLAB Function/4(Mx_ctrl) -> Scope3/1, Simulink-PS Converter8/1
  MATLAB Function/5(My_ctrl) -> Scope4/1, Simulink-PS Converter9/1
  MATLAB Function/6(Mz_ctrl) -> Simulink-PS Converter10/1
  MATLAB Function/3(Tz_ctrl) -> Scope2/1, Simulink-PS Converter7/1
  omega1/1 -> MATLAB Function/1(omega1)
  omega2/1 -> MATLAB Function/2(omega2)
  alfa1/1 -> MATLAB Function/3(alfa1)
  alfa2/1 -> MATLAB Function/4(alfa2)
  connections:
  External Force and Torque/RConn1 -- Conn1/RConn1
  Simulink-PS Converter5/RConn1 -- External Force and Torque/LConn1
  Simulink-PS Converter6/RConn1 -- External Force and Torque/LConn2
  Simulink-PS Converter7/RConn1 -- External Force and Torque/LConn3
  Simulink-PS Converter8/RConn1 -- External Force and Torque/LConn4
  Simulink-PS Converter9/RConn1 -- External Force and Torque/LConn5
  Simulink-PS Converter10/RConn1 -- External Force and Torque/LConn6

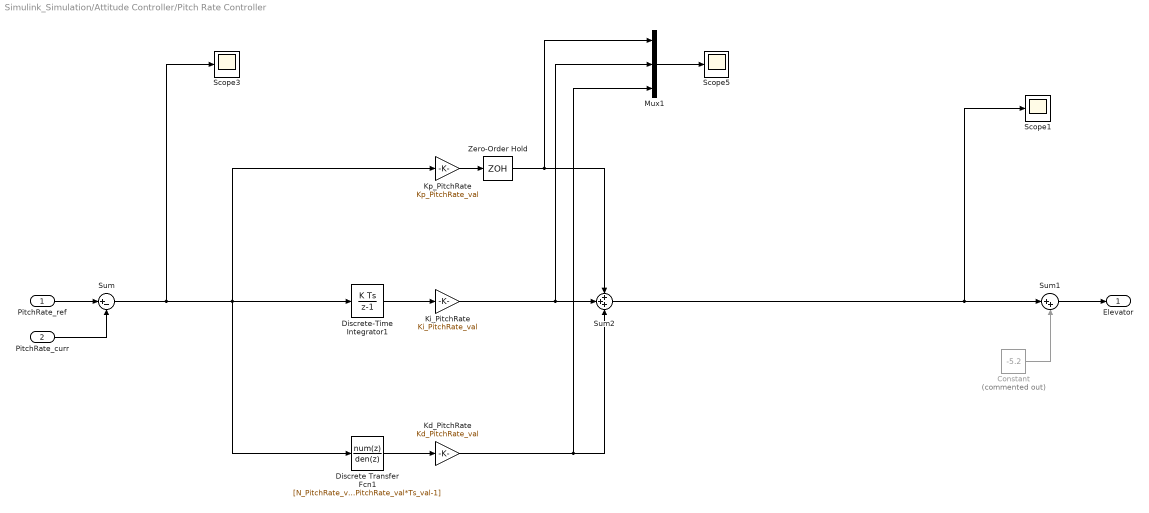
== system Simulink_Simulation/Attitude Controller/Pitch Rate Controller ==
  PitchRate_ref : Inport
  PitchRate_curr : Inport  Port=2
  Constant : Constant  Commented=on  Value=-5.2
  Discrete Transfer Fcn1 : DiscreteTransferFcn  Numerator=[N_PitchRate_val, -N_PitchRate_val]  Denominator=[1, N_PitchRate_val*Ts_val-1]  SampleTime=Ts_val
  Discrete-Time Integrator1 : DiscreteIntegrator  SampleTime=Ts_val  ICPrevOutput=DiscIntNeverNeededParam  ICPrevScaledInput=DiscIntNeverNeededParam
  Kd_PitchRate : Gain  Gain=Kd_PitchRate_val
  Ki_PitchRate : Gain  Gain=Ki_PitchRate_val
  Kp_PitchRate : Gain  Gain=Kp_PitchRate_val
  Mux1 : Mux  Inputs=3
  Scope1 : Scope
  Scope3 : Scope
  Scope5 : Scope
  Sum : Sum  Inputs=|+-
  Sum1 : Sum  Inputs=|++
  Sum2 : Sum  Inputs=+++
  Zero-Order Hold : ZeroOrderHold  SampleTime=Ts_val
  Elevator : Outport
  wires:
  Ki_PitchRate/1 -> Mux1/2, Sum2/2
  Mux1/1 -> Scope5/1
  Kd_PitchRate/1 -> Sum2/3, Mux1/3
  Discrete-Time Integrator1/1 -> Ki_PitchRate/1
  Discrete Transfer Fcn1/1 -> Kd_PitchRate/1
  Sum2/1 -> Scope1/1, Sum1/1
  Kp_PitchRate/1 -> Zero-Order Hold/1
  Zero-Order Hold/1 -> Mux1/1, Sum2/1
  Sum/1 -> Scope3/1, Discrete-Time Integrator1/1, Discrete Transfer Fcn1/1, Kp_PitchRate/1
  PitchRate_ref/1 -> Sum/1
  PitchRate_curr/1 -> Sum/2
  Sum1/1 -> Elevator/1
  Constant/1 -> Sum1/2

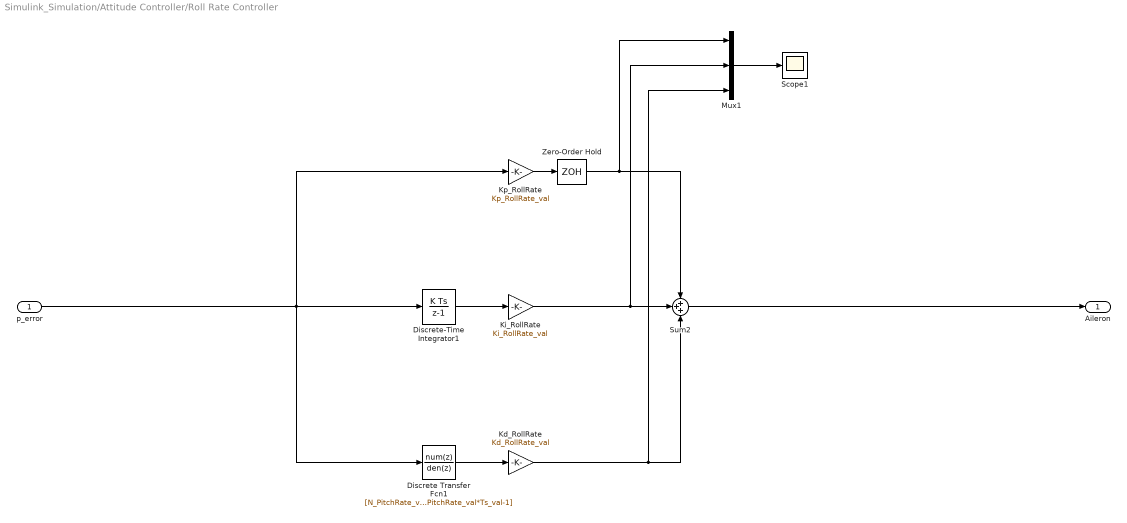
== system Simulink_Simulation/Attitude Controller/Roll Rate Controller ==
  p_error : Inport
  Discrete Transfer Fcn1 : DiscreteTransferFcn  Numerator=[N_PitchRate_val, -N_PitchRate_val]  Denominator=[1, N_PitchRate_val*Ts_val-1]  SampleTime=Ts_val
  Discrete-Time Integrator1 : DiscreteIntegrator  SampleTime=Ts_val  ICPrevOutput=DiscIntNeverNeededParam  ICPrevScaledInput=DiscIntNeverNeededParam
  Kd_RollRate : Gain  Gain=Kd_RollRate_val
  Ki_RollRate : Gain  Gain=Ki_RollRate_val
  Kp_RollRate : Gain  Gain=Kp_RollRate_val
  Mux1 : Mux  Inputs=3
  Scope1 : Scope
  Sum2 : Sum  Inputs=+++
  Zero-Order Hold : ZeroOrderHold  SampleTime=Ts_val
  Aileron : Outport
  wires:
  p_error/1 -> Discrete Transfer Fcn1/1, Kp_RollRate/1, Discrete-Time Integrator1/1
  Kp_RollRate/1 -> Zero-Order Hold/1
  Kd_RollRate/1 -> Sum2/3, Mux1/3
  Sum2/1 -> Aileron/1
  Zero-Order Hold/1 -> Mux1/1, Sum2/1
  Discrete-Time Integrator1/1 -> Ki_RollRate/1
  Mux1/1 -> Scope1/1
  Ki_RollRate/1 -> Mux1/2, Sum2/2
  Discrete Transfer Fcn1/1 -> Kd_RollRate/1

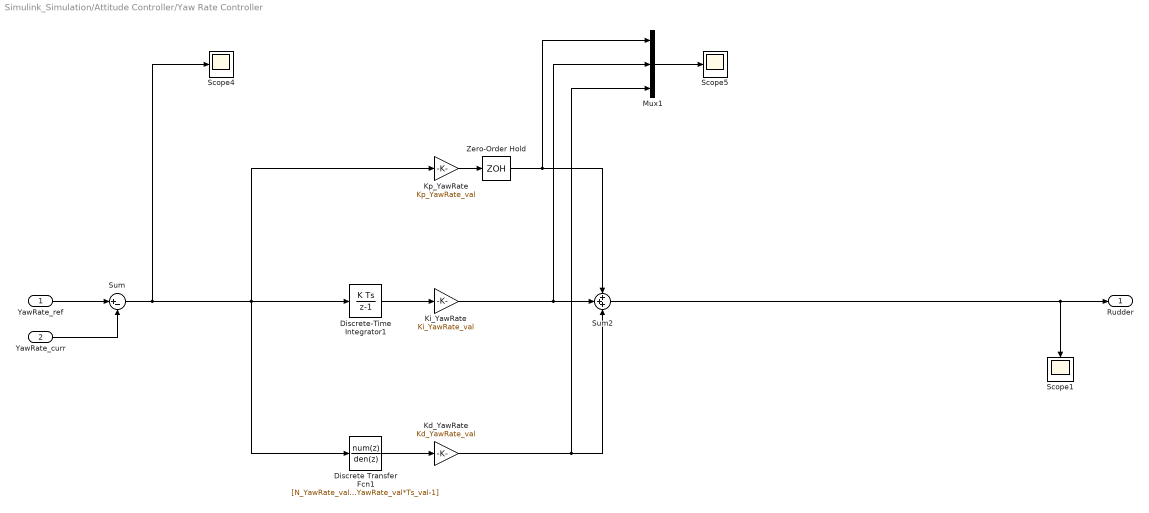
== system Simulink_Simulation/Attitude Controller/Yaw Rate Controller ==
  YawRate_ref : Inport
  YawRate_curr : Inport  Port=2
  Discrete Transfer Fcn1 : DiscreteTransferFcn  Numerator=[N_YawRate_val, -N_YawRate_val]  Denominator=[1, N_YawRate_val*Ts_val-1]  SampleTime=Ts_val
  Discrete-Time Integrator1 : DiscreteIntegrator  SampleTime=Ts_val  ICPrevOutput=DiscIntNeverNeededParam  ICPrevScaledInput=DiscIntNeverNeededParam
  Kd_YawRate : Gain  Gain=Kd_YawRate_val
  Ki_YawRate : Gain  Gain=Ki_YawRate_val
  Kp_YawRate : Gain  Gain=Kp_YawRate_val
  Mux1 : Mux  Inputs=3
  Scope1 : Scope
  Scope4 : Scope
  Scope5 : Scope
  Sum : Sum  Inputs=|+-
  Sum2 : Sum  Inputs=+++
  Zero-Order Hold : ZeroOrderHold  SampleTime=Ts_val
  Rudder : Outport
  wires:
  Kp_YawRate/1 -> Zero-Order Hold/1
  Kd_YawRate/1 -> Sum2/3, Mux1/3
  Zero-Order Hold/1 -> Mux1/1, Sum2/1
  Discrete-Time Integrator1/1 -> Ki_YawRate/1
  Discrete Transfer Fcn1/1 -> Kd_YawRate/1
  Mux1/1 -> Scope5/1
  Ki_YawRate/1 -> Mux1/2, Sum2/2
  Sum2/1 -> Rudder/1, Scope1/1
  YawRate_ref/1 -> Sum/1
  Sum/1 -> Scope4/1, Discrete-Time Integrator1/1, Discrete Transfer Fcn1/1, Kp_YawRate/1
  YawRate_curr/1 -> Sum/2

== system Simulink_Simulation/Aircraft Dynamics/Subsystem/P_PWR_Nozzle_1_RIGID ==
  ReferenceFrame : sm_lib/Frames and Transforms/Reference Frame
  Solid : sm_lib/Body Elements/File Solid  ExtGeomFileName=#P_PWR_Nozzle_Predeterminado_sldprt.STEP  UnitType=FromFile  ExtGeomFileUnits=m  StepReaderType=HEX  ExportConvexHullGeometry=off  InertiaType=Custom  Mass=smiData.Solid(2).mass  MassUnits=kg  CenterOfMass=smiData.Solid(2).CoM  CenterOfMassUnits=mm  MomentsOfInertia=smiData.Solid(2).MoI  MomentsOfInertiaUnits=kg*mm^2  ProductsOfInertia=smiData.Solid(2).PoI  ProductsOfInertiaUnits=kg*mm^2  BasedOnType=DensityFromFile  Density=1000  DensityUnits=kg/m^3  DoExposeReferenceFrame=on  SerializedFrames=<Frames/>  GraphicType=FromGeometry  MarkerShape=Sphere  MarkerSize=10  GraphicVisPropType=SimpleVisualProperties  GraphicDiffuseColor=smiData.Solid(2).color  GraphicSpecularColor=[0.5 0.5 0.5 1.0]  GraphicAmbientColor=[0.15 0.15 0.15 1.0]  GraphicEmissiveColor=[0.0 0.0 0.0 1.0]  GraphicShininess=75  GraphicOpacity=smiData.Solid(2).opacity
  Transform : sm_lib/Frames and Transforms/Rigid Transform  TranslationMethod=Cartesian  TranslationStandardOffset=0  TranslationLengthUnit=mm  TranslationStandardAxis=+Z  TranslationCartesianOffset=smiData.RigidTransform(2).translation  TranslationROffset=0  TranslationROffsetUnits=m  TranslationZOffset=0  TranslationZOffsetUnits=m  TranslationThetaOffset=0  TranslationThetaOffsetUnits=deg  RotationMethod=ArbitraryAxis  RotationAngleUnits=rad  RotationStandardAxis=+Z  RotationAngle=smiData.RigidTransform(2).angle  RotationArbitraryAxis=smiData.RigidTransform(2).axis  FollAlignAxisA=+X  BaseAlignAxisA=+Y  FollAlignAxisB=+Y  BaseAlignAxisB=+Z  RotationSequenceAxes=FollowerAxes  RotationSequence=XYX  RotationSequenceAngles=[0 0 0]  RotationSequenceAnglesUnits=deg  RotationMatrix=[1 0 0; 0 1 0; 0 0 1]  Quaternion=[1 0 0 0]
  F : PMIOPort  Side=Left
  connections:
  Solid/RConn1 -- ReferenceFrame/RConn1 -- Transform/LConn1
  Transform/RConn1 -- F/RConn1

== system Simulink_Simulation/Aircraft Dynamics/Subsystem/P_PWR_Nozzle_2_RIGID ==
  ReferenceFrame : sm_lib/Frames and Transforms/Reference Frame
  Solid : sm_lib/Body Elements/File Solid  ExtGeomFileName=#P_PWR_Nozzle_Predeterminado_sldprt.STEP  UnitType=FromFile  ExtGeomFileUnits=m  StepReaderType=HEX  ExportConvexHullGeometry=off  InertiaType=Custom  Mass=smiData.Solid(2).mass  MassUnits=kg  CenterOfMass=smiData.Solid(2).CoM  CenterOfMassUnits=mm  MomentsOfInertia=smiData.Solid(2).MoI  MomentsOfInertiaUnits=kg*mm^2  ProductsOfInertia=smiData.Solid(2).PoI  ProductsOfInertiaUnits=kg*mm^2  BasedOnType=DensityFromFile  Density=1000  DensityUnits=kg/m^3  DoExposeReferenceFrame=on  SerializedFrames=<Frames/>  GraphicType=FromGeometry  MarkerShape=Sphere  MarkerSize=10  GraphicVisPropType=SimpleVisualProperties  GraphicDiffuseColor=smiData.Solid(2).color  GraphicSpecularColor=[0.5 0.5 0.5 1.0]  GraphicAmbientColor=[0.15 0.15 0.15 1.0]  GraphicEmissiveColor=[0.0 0.0 0.0 1.0]  GraphicShininess=75  GraphicOpacity=smiData.Solid(2).opacity
  Transform : sm_lib/Frames and Transforms/Rigid Transform  TranslationMethod=Cartesian  TranslationStandardOffset=0  TranslationLengthUnit=mm  TranslationStandardAxis=+Z  TranslationCartesianOffset=smiData.RigidTransform(4).translation  TranslationROffset=0  TranslationROffsetUnits=m  TranslationZOffset=0  TranslationZOffsetUnits=m  TranslationThetaOffset=0  TranslationThetaOffsetUnits=deg  RotationMethod=ArbitraryAxis  RotationAngleUnits=rad  RotationStandardAxis=+Z  RotationAngle=smiData.RigidTransform(4).angle  RotationArbitraryAxis=smiData.RigidTransform(4).axis  FollAlignAxisA=+X  BaseAlignAxisA=+Y  FollAlignAxisB=+Y  BaseAlignAxisB=+Z  RotationSequenceAxes=FollowerAxes  RotationSequence=XYX  RotationSequenceAngles=[0 0 0]  RotationSequenceAnglesUnits=deg  RotationMatrix=[1 0 0; 0 1 0; 0 0 1]  Quaternion=[1 0 0 0]
  F : PMIOPort  Side=Left
  connections:
  Solid/RConn1 -- ReferenceFrame/RConn1 -- Transform/LConn1
  Transform/RConn1 -- F/RConn1
